simulink model "busCreators01"  (R2025b)
settings: Solver=VariableStepAuto  StartTime=0.0  StopTime=10.0  RelTol=1e-3
settings Model: Creator=gdudgeon  LastModifiedBy=gdudgeon
settings RTWCC: GPUComputeCapability=3.5

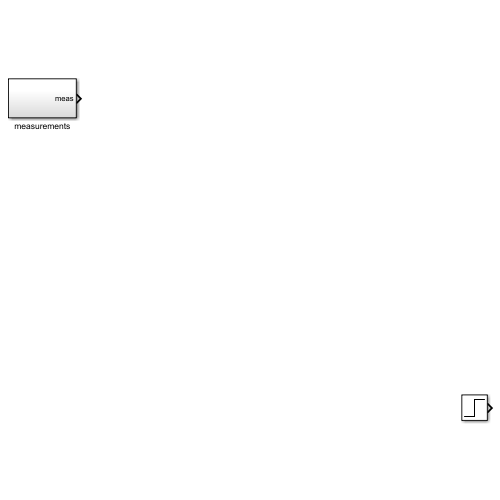
[thumbnail: Simulink's stored preview of the top-level diagram]
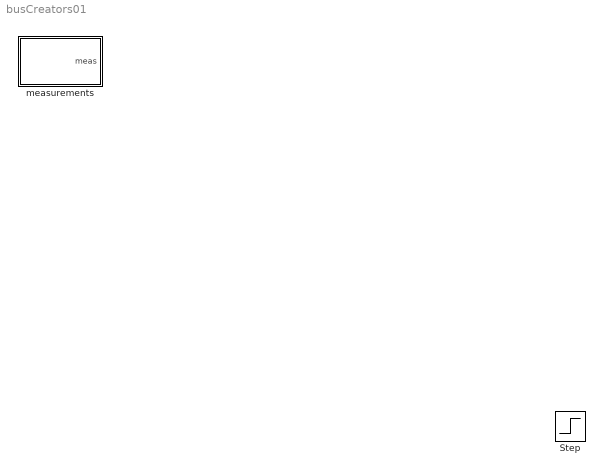
== system busCreators01 ==
  Step : Step  SampleTime=0
  measurements : Subsystem

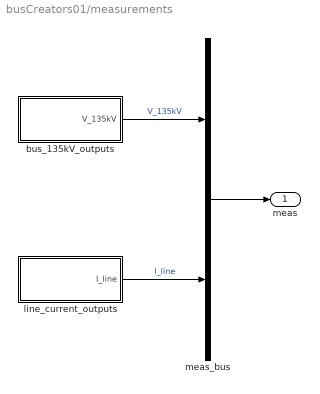
== system busCreators01/measurements ==
  bus_135kV_outputs : Subsystem
  line_current_outputs : Subsystem
  meas_bus : BusCreator  Inputs=2
  meas : Outport
  wires:
  bus_135kV_outputs/1(V_135kV) -> meas_bus/1  "V_135kV"
  line_current_outputs/1(I_line) -> meas_bus/2  "I_line"
  meas_bus/1 -> meas/1

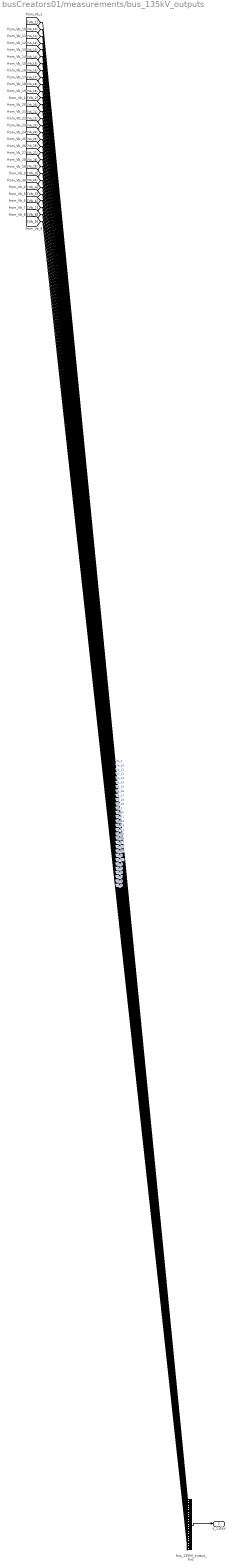
== system busCreators01/measurements/bus_135kV_outputs ==
  bus_135kV_output_bus : BusCreator  Inputs=30
  V_135kV : Outport  OutDataTypeStr=Bus: n_slBus1  VectorParamsAs1DForOutWhenUnconnected=off
  wires:
  [Vb_9] -> bus_135kV_output_bus/30  "Vb_9"
  [Vb_8] -> bus_135kV_output_bus/29  "Vb_8"
  [Vb_7] -> bus_135kV_output_bus/28  "Vb_7"
  [Vb_6] -> bus_135kV_output_bus/27  "Vb_6"
  [Vb_5] -> bus_135kV_output_bus/26  "Vb_5"
  [Vb_4] -> bus_135kV_output_bus/25  "Vb_4"
  [Vb_30] -> bus_135kV_output_bus/24  "Vb_30"
  [Vb_3] -> bus_135kV_output_bus/23  "Vb_3"
  [Vb_29] -> bus_135kV_output_bus/22  "Vb_29"
  [Vb_28] -> bus_135kV_output_bus/21  "Vb_28"
  [Vb_27] -> bus_135kV_output_bus/20  "Vb_27"
  [Vb_26] -> bus_135kV_output_bus/19  "Vb_26"
  [Vb_25] -> bus_135kV_output_bus/18  "Vb_25"
  [Vb_24] -> bus_135kV_output_bus/17  "Vb_24"
  [Vb_23] -> bus_135kV_output_bus/16  "Vb_23"
  [Vb_22] -> bus_135kV_output_bus/15  "Vb_22"
  [Vb_21] -> bus_135kV_output_bus/14  "Vb_21"
  [Vb_20] -> bus_135kV_output_bus/13  "Vb_20"
  [Vb_2] -> bus_135kV_output_bus/12  "Vb_2"
  [Vb_19] -> bus_135kV_output_bus/11  "Vb_19"
  [Vb_18] -> bus_135kV_output_bus/10  "Vb_18"
  [Vb_17] -> bus_135kV_output_bus/9  "Vb_17"
  [Vb_16] -> bus_135kV_output_bus/8  "Vb_16"
  [Vb_15] -> bus_135kV_output_bus/7  "Vb_15"
  [Vb_14] -> bus_135kV_output_bus/6  "Vb_14"
  [Vb_13] -> bus_135kV_output_bus/5  "Vb_13"
  [Vb_12] -> bus_135kV_output_bus/4  "Vb_12"
  [Vb_11] -> bus_135kV_output_bus/3  "Vb_11"
  [Vb_10] -> bus_135kV_output_bus/2  "Vb_10"
  [Vb_1] -> bus_135kV_output_bus/1  "Vb_1"
  bus_135kV_output_bus/1 -> V_135kV/1

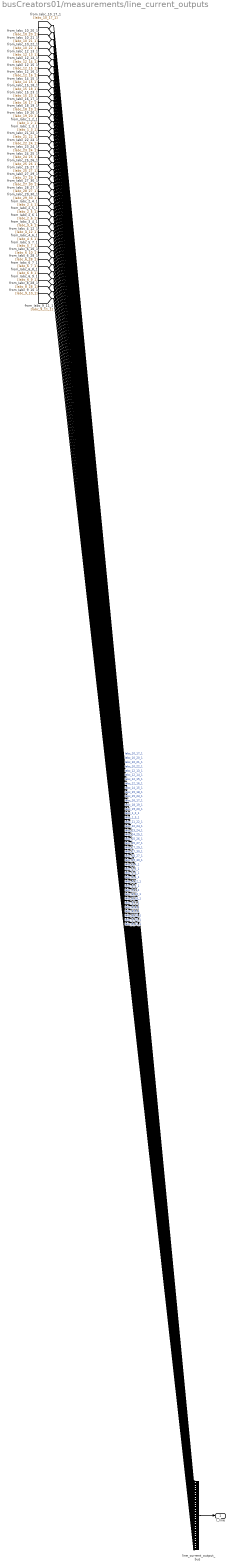
== system busCreators01/measurements/line_current_outputs ==
  line_current_output_bus : BusCreator  Inputs=41
  I_line : Outport  OutDataTypeStr=Bus: n_slBus2  VectorParamsAs1DForOutWhenUnconnected=off
  wires:
  [Iabc_9_11_1] -> line_current_output_bus/41  "Iabc_9_11_1"
  [Iabc_9_10_1] -> line_current_output_bus/40  "Iabc_9_10_1"
  [Iabc_8_28_1] -> line_current_output_bus/39  "Iabc_8_28_1"
  [Iabc_6_9_1] -> line_current_output_bus/38  "Iabc_6_9_1"
  [Iabc_6_8_1] -> line_current_output_bus/37  "Iabc_6_8_1"
  [Iabc_6_7_1] -> line_current_output_bus/36  "Iabc_6_7_1"
  [Iabc_6_28_1] -> line_current_output_bus/35  "Iabc_6_28_1"
  [Iabc_6_10_1] -> line_current_output_bus/34  "Iabc_6_10_1"
  [Iabc_5_7_1] -> line_current_output_bus/33  "Iabc_5_7_1"
  [Iabc_4_6_1] -> line_current_output_bus/32  "Iabc_4_6_1"
  [Iabc_4_12_1] -> line_current_output_bus/31  "Iabc_4_12_1"
  [Iabc_3_4_1] -> line_current_output_bus/30  "Iabc_3_4_1"
  [Iabc_2_6_1] -> line_current_output_bus/29  "Iabc_2_6_1"
  [Iabc_2_5_1] -> line_current_output_bus/28  "Iabc_2_5_1"
  [Iabc_2_4_1] -> line_current_output_bus/27  "Iabc_2_4_1"
  [Iabc_29_30_1] -> line_current_output_bus/26  "Iabc_29_30_1"
  [Iabc_28_27_1] -> line_current_output_bus/25  "Iabc_28_27_1"
  [Iabc_27_30_1] -> line_current_output_bus/24  "Iabc_27_30_1"
  [Iabc_27_29_1] -> line_current_output_bus/23  "Iabc_27_29_1"
  [Iabc_25_27_1] -> line_current_output_bus/22  "Iabc_25_27_1"
  [Iabc_25_26_1] -> line_current_output_bus/21  "Iabc_25_26_1"
  [Iabc_24_25_1] -> line_current_output_bus/20  "Iabc_24_25_1"
  [Iabc_23_24_1] -> line_current_output_bus/19  "Iabc_23_24_1"
  [Iabc_22_24_1] -> line_current_output_bus/18  "Iabc_22_24_1"
  [Iabc_21_22_1] -> line_current_output_bus/17  "Iabc_21_22_1"
  [Iabc_1_3_1] -> line_current_output_bus/16  "Iabc_1_3_1"
  [Iabc_1_2_1] -> line_current_output_bus/15  "Iabc_1_2_1"
  [Iabc_19_20_1] -> line_current_output_bus/14  "Iabc_19_20_1"
  [Iabc_18_19_1] -> line_current_output_bus/13  "Iabc_18_19_1"
  [Iabc_16_17_1] -> line_current_output_bus/12  "Iabc_16_17_1"
  [Iabc_15_23_1] -> line_current_output_bus/11  "Iabc_15_23_1"
  [Iabc_15_18_1] -> line_current_output_bus/10  "Iabc_15_18_1"
  [Iabc_14_15_1] -> line_current_output_bus/9  "Iabc_14_15_1"
  [Iabc_12_16_1] -> line_current_output_bus/8  "Iabc_12_16_1"
  [Iabc_12_15_1] -> line_current_output_bus/7  "Iabc_12_15_1"
  [Iabc_12_14_1] -> line_current_output_bus/6  "Iabc_12_14_1"
  [Iabc_12_13_1] -> line_current_output_bus/5  "Iabc_12_13_1"
  [Iabc_10_22_1] -> line_current_output_bus/4  "Iabc_10_22_1"
  [Iabc_10_21_1] -> line_current_output_bus/3  "Iabc_10_21_1"
  [Iabc_10_20_1] -> line_current_output_bus/2  "Iabc_10_20_1"
  [Iabc_10_17_1] -> line_current_output_bus/1  "Iabc_10_17_1"
  line_current_output_bus/1 -> I_line/1
